simulink model "Cv_4"  (R2022a)
settings: Solver=VariableStepAuto  StartTime=0.0  StopTime=2  MaxStep=1e-3  RelTol=1e-3
values from neighbouring files (symbols this model uses):
  cfi = 0.1    [Cv_4_params.m]
  I = 1e-4    (= 0.0001)    [Cv_4_params.m]
  L = 5e-3    (= 0.005)    [Cv_4_params.m]
  Mz = 0.02*0    (= 0)    [Cv_4_params.m]
  R = 20    [Cv_4_params.m]
  U = 12    [Cv_4_params.m]
settings Model: Creator=221208  LastModifiedBy=221208

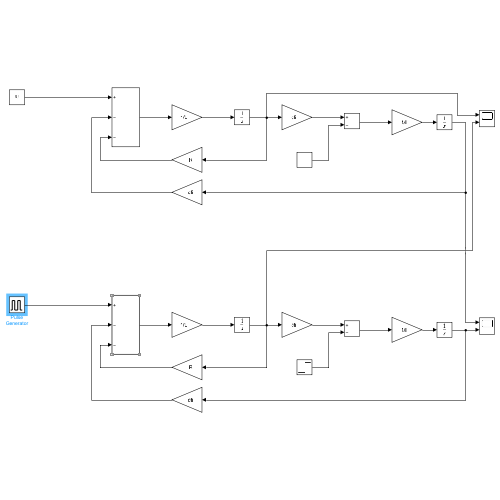
[thumbnail: Simulink's stored preview of the top-level diagram]
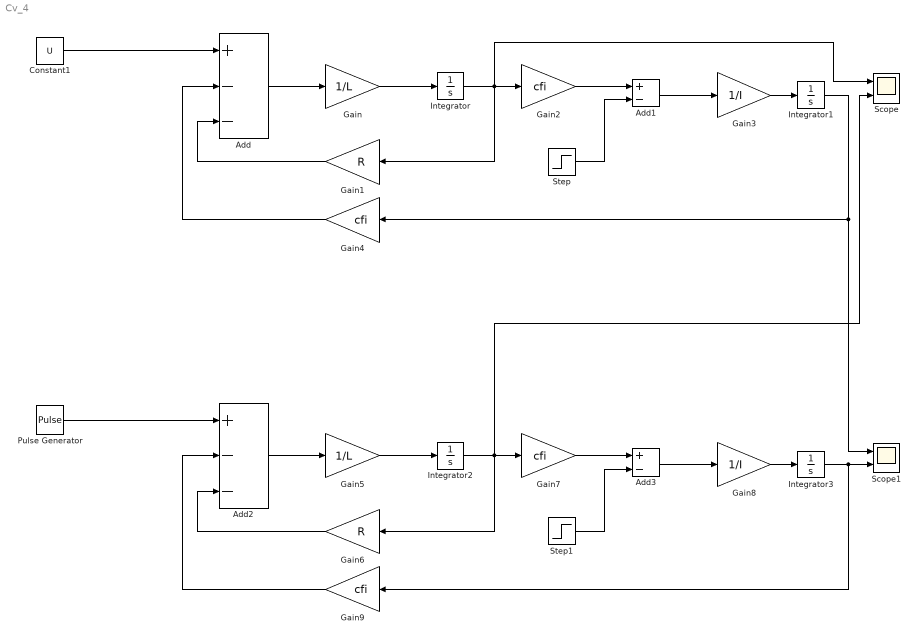
== system Cv_4 ==
  Add : Sum  Inputs=+--
  Add1 : Sum  Inputs=+-
  Add2 : Sum  Inputs=+--
  Add3 : Sum  Inputs=+-
  Constant1 : Constant  Value=U
  Gain : Gain  Gain=1/L
  Gain1 : Gain  Gain=R
  Gain{2,4,7,9} (4 alike) : Gain  Gain=cfi
  Gain3 : Gain  Gain=1/I
  Gain5 : Gain  Gain=1/L
  Gain6 : Gain  Gain=R
  Gain8 : Gain  Gain=1/I
  Integrator{,1..3} (4 alike) : Integrator
  Pulse Generator : DiscretePulseGenerator  PulseType=Time based  Amplitude=U  Period=1/10000  PulseWidth=50
  Scope : Scope  NumInputPorts=2
  Scope1 : Scope  NumInputPorts=2
  Step : Step  After=Mz  SampleTime=0
  Step1 : Step  After=Mz  SampleTime=0
  wires:
  Gain/1 -> Integrator/1
  Add/1 -> Gain/1
  Constant1/1 -> Add/1
  Integrator/1 -> Scope/1, Gain1/1, Gain2/1
  Gain1/1 -> Add/3
  Gain2/1 -> Add1/1
  Step/1 -> Add1/2
  Gain3/1 -> Integrator1/1
  Add1/1 -> Gain3/1
  Gain4/1 -> Add/2
  Integrator1/1 -> Scope1/1, Gain4/1
  Gain9/1 -> Add2/2
  Integrator3/1 -> Gain9/1, Scope1/2
  Gain8/1 -> Integrator3/1
  Gain6/1 -> Add2/3
  Pulse Generator/1 -> Add2/1
  Integrator2/1 -> Scope/2, Gain6/1, Gain7/1
  Step1/1 -> Add3/2
  Add2/1 -> Gain5/1
  Add3/1 -> Gain8/1
  Gain7/1 -> Add3/1
  Gain5/1 -> Integrator2/1
